simulink model "sdl_vehicle_starter"  (Simulink 7.9)
settings: Solver=ode23t  StartTime=0.0  StopTime=150  FixedStep=1e-3  RelTol=1e-4
model workspace (MAT data in the model file):
  vi = Simulink.Parameter
  vi.Value = 960
  vi.DataType = 'auto'
PreLoadFcn:
  | num_fric_surf = 6;
  | eff_tor_rad = 0.4;
  | engagement_area = 0.0025;
  | peak_normal = 0.55;
  | fric_coeff = 0.5;
  | clutchRise = 0.1;
  | velTol = 1e-3;
  | pressThresh = 0.05;
  | p0 = 20e5;
undefined symbols (not defined in the file): sigbuilder_block
libraries: fl_lib x20, nesl_utility x14, sdl_lib x12
Description:
  | Vehicle With Automatic Transmission
  | 
  | This example shows a complete vehicle with SimDriveline(TM) blocks, from
  | engine, drivetrain, and transmission, to tire and vehicle dynamics. The
  | transmission controller is preprogrammed, but can be changed to respond to
  | engine and vehicle behavior.
  | 
  | 
  | 
  | 
  | 
  | Copyright 2008-2012 The MathWorks, Inc.
CloseFcn:
  | clear num_fric_surf eff_tor_rad engagement_area
  | clear peak_normal fric_coeff clutchRise
  | clear velTol pressThresh p0
settings Model: FPTRunName=Active  Creator=MathWorks  LastModifiedBy=sbiagion  ExtModeAutoUpdateStatusClock=off
settings SolverCC: ZcThreshold=0  ZeroCrossAlgorithm=Adaptive
settings DataIOCC: SaveOutput=off  SignalLogging=off  DSMLogging=off  SaveTime=off  SignalLoggingName=logsOut
settings OptimizationCC: InitFltsAndDblsToZero=on
settings DebuggingCC: AlgebraicLoopMsg=none  SaveWithParameterizedLinksMsg=none  CheckExecutionContextPreStartOutputMsg=on  CheckExecutionContextRuntimeOutputMsg=on  SignalResolutionControl=TryResolveAllWithWarning  MaskedZcDiagnostic=none  SolverPrmCheckMsg=none  MultiTaskDSMMsg=warning  MultiTaskCondExecSysMsg=none  SigSpecEnsureSampleTimeMsg=none  StrictBusMsg=None
settings HardwareCC: TargetEndianess=LittleEndian  TargetHWDeviceType=MATLAB Host  ProdEqTarget=off
settings ModelReferenceCC: UpdateModelReferenceTargets=IfOutOfDate
settings RTWCC: ProcessScript=grt_make_rtw_hook  IncludeERTFirstTime=on
settings CodeAppCC: CustomSymbolStrType=$N$R$M_T
settings GRTTargetCC: CombineOutputUpdateFcns=off  GRTInterface=on

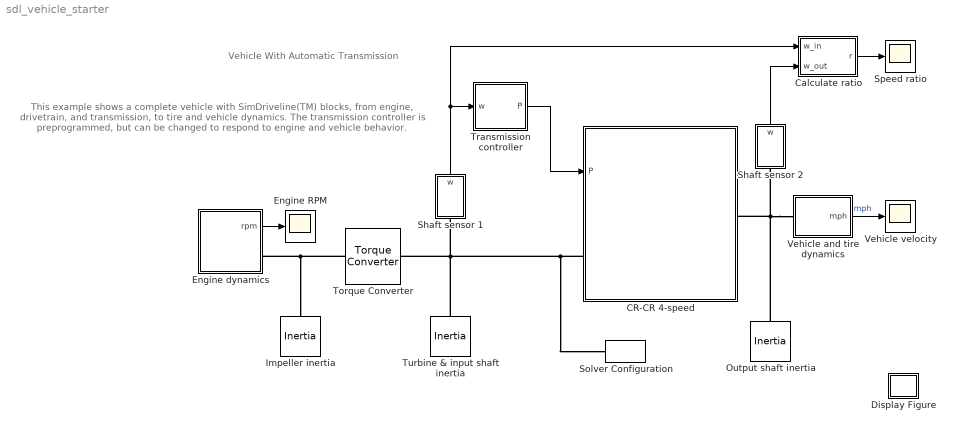
== system sdl_vehicle_starter ==
  note: Vehicle With Automatic Transmission
  note: This example shows a complete vehicle
      | with SimDriveline(TM) blocks, from
      | engine, drivetrain, and transmission, to
      | tire and vehicle dynamics. The
      | transmission controller is
      | preprogrammed, but can be changed to
      | respond to engine and vehicle behavior.
  CR-CR 4-speed : Subsystem  mask(CR-CR 4-Speed){}
      mask help: This is a template for a CR-CR 4-speed transmission. Copy it to your model, open it as a subsystem, and modify it for your use.
      mask init:
      | drive_preinitmask(); Icon = drive_crcrgearblock('Mask');
      settings: OpenFcn=open_system(gcbh,'force');
      mask Help: web(drive_help);
      mask Display:
      | plot(Icon.x1,Icon.y1);
      | plot(Icon.x1_1,Icon.y1_1);
      | plot(Icon.x2,Icon.y2);
      | plot(Icon.x3,Icon.y3);
      | plot(Icon.x3_1,Icon.y3_1);
      | plot(Icon.x4,Icon.y4);
      | plot(Icon.x5,Icon.y5);
      | plot(Icon.x6,Icon.y6);
      | plot(Icon.x7,Icon.y7);
      | plot(Icon.x8,Icon.y8);
      | plot(Icon.x9,Icon.y9);
      | plot(Icon.x10,Icon.y10);
      | plot(Icon.x11,Icon.y11);
      | plot(Icon.x12,Icon.y12);
      | plot(Icon.x13,Icon.y13);
      | plot(Icon.x14,Icon.y14);
      | plot(Icon.x15,Icon.y15);
      | plot(Icon.x16,Icon.y16);
      | plot(Icon.x16_1,Icon.y16_1);
      | plot(Icon.x16_2,Icon.y16_2);
      | plot(Icon.x17,Icon.y17);
      | plot(Icon.x18,Icon.y18);
      | plot(Icon.x18_1,Icon.y18_1);
      | plot(Icon.x18_2,Icon.y18_2);
      | plot(Icon.x19,Icon.y19);
      | plot(Icon.x20,Icon.y20);
      | plot(Icon.x21,Icon.y21);
      | plot(Icon.x22,Icon.y22);
      | plot(Icon.x23,Icon.y23);
      | plot(Icon.x24,Icon.y24);
      | plot(Icon.x25,Icon.y25);
      | plot(Icon.x26,Icon.y26);
      | plot(Icon.x27,Icon.y27);
      | plot(Icon.x28,Icon.y28);
      | plot(Icon.x29,Icon.y29);
      | 
      | plot(Icon.LowerLeftx,Icon.LowerLefty);
      | plot(Icon.UpperRightx,Icon.UpperRighty);
  Calculate ratio : Subsystem
  Display Figure : Subsystem  Description=Help callback for CR-CR transmission model: sdl_vehicle.mdl
      settings: OpenFcn=helpview([docroot '/toolbox/physmod/sdl/sdl.map'], 'sdl_vehicle_help');
      mask Type: Help callback
      mask Display: image(imread('info.bmp'))
  Engine RPM : Scope
      settings: TimeRange=150  YMin=500  YMax=4000  MaxDataPoints=500000  SampleTime=0.1
  Engine dynamics : Subsystem
  Impeller inertia : fl_lib/Mechanical/Rotational Elements/Inertia  inertia=0.02 kg*m^2  initial_velocity=vi rpm  t_Log=off  LocalVarNames=|t  LocalVarDescs=|t  LocalVarLogging=0
  Output shaft inertia : fl_lib/Mechanical/Rotational Elements/Inertia  inertia=1e-1 kg*m^2  initial_velocity=0 rad/s  t_Log=off  LocalVarNames=|t  LocalVarDescs=|t  LocalVarLogging=0
  Shaft sensor 1 : Subsystem
  Shaft sensor 2 : Subsystem
  Solver Configuration : nesl_utility/Solver Configuration  PhysicalDomain=network_engine_domain  LeftPortType=input  RightPortType=generic  SubClassName=solver  UseCustomDae=off  DoDC=off  ResidualTolerance=1e-9  UseLocalSolver=off  LocalSolverChoice=NE_BACKWARD_EULER_ADVANCER  LocalSolverSampleTime=0.001  DoFixedCost=off  MaxNonlinIter=3  MaxModeIter=2  LinearAlgebra=Sparse  Accelerate=off  Profile=off  UseLocalSampling=off  DelaysMemoryBudget=1024
  Speed ratio : Scope
      settings: TimeRange=150  YMin=0  YMax=1.5  SaveName=ScopeData5  MaxDataPoints=500000  SampleTime=0.1
  Torque Converter : sdl_lib/Couplings & Drives/Torque Converter  n_vector=[0 0.50 0.60 0.70 0.80 0.87 0.92 0.94 0.96 0.97]  trq_vector=[2.2320 1.5462 1.4058 1.2746 1.1528 1.0732 1.0192 0.9983 0.9983 0.9983]  cf_vector_parameterization=1  cf_vector_reference_speed=1  cf_vector=[12.2938 12.8588 13.1452 13.6285 14.6163 16.2675 19.3503 22.1046 29.9986 50.00] (rad/s)/(N*m)^0.5  cf_vector_sq=1e-3*[ 6.616 6.048 5.787 5.384 4.681 3.779 2.671 2.047 1.111 0.400] N*m/(rad/s)^2  interp_method=1  extrap_method=1  model_lag=0  tau=0.02 s  initial_trq_ratio=0  trq_imp_s_Log=off  trq_imp_Log=off  torque_ratio_Log=off  trq_ratio_inst_Log=off  trq_trb_Log=off  w_imp_Log=off  w_trb_Log=off  power_imp_Log=off  power_trb_Log=off  power_loss_Log=off  efficiency_Log=off  LocalVarNames=|trq_imp_s|trq_imp|N_t|trq_ratio_inst|trq_trb|w_imp|w_trb|power_imp|power_trb|power_loss|efficiency  LocalVarDescs=|Static torque on impeller shaft (N*m)|Transient torque on impeller shaft (N*m)|Static torque ratio|Instant torque ratio|Torque on turbine shaft (N*m)|Angular velocity of impeller shaft (rad/s)|Angular velocity of turbine shaft (rad/s)|Power on impeller shaft (W)|Power on turbine shaft (W)|Power loss (W)|Efficiency)  LocalVarLogging=[0 0 0 0 0 0 0 0 0 0 0]
  Transmission controller : Subsystem
  Turbine & input shaft inertia : fl_lib/Mechanical/Rotational Elements/Inertia  inertia=1e-2 kg*m^2  initial_velocity=0 rad/s  t_Log=off  LocalVarNames=|t  LocalVarDescs=|t  LocalVarLogging=0
  Vehicle velocity : Scope
      settings: YMin=0  YMax=120  SaveName=ScopeData2  MaxDataPoints=500000  SampleTime=0.1
  Vehicle and tire dynamics : Subsystem
  wires:
  Shaft sensor 1/1(w) -> Calculate ratio/1(w_in), Transmission controller/1(w)
  Transmission controller/1(P) -> CR-CR 4-speed/1(P)
  Shaft sensor 2/1(w) -> Calculate ratio/2(w_out)
  Calculate ratio/1(r) -> Speed ratio/1
  Vehicle and tire dynamics/1(mph) -> Vehicle velocity/1  "mph"
  Engine dynamics/1(rpm) -> Engine RPM/1
  connections:
  Torque Converter/RConn1 -- Shaft sensor 1/LConn1 -- Turbine & input shaft inertia/LConn1 -- CR-CR 4-speed/LConn1 -- Solver Configuration/RConn1
  Vehicle and tire dynamics/LConn1 -- Shaft sensor 2/LConn1 -- Output shaft inertia/LConn1 -- CR-CR 4-speed/RConn1
  Engine dynamics/RConn1 -- Impeller inertia/LConn1 -- Torque Converter/LConn1

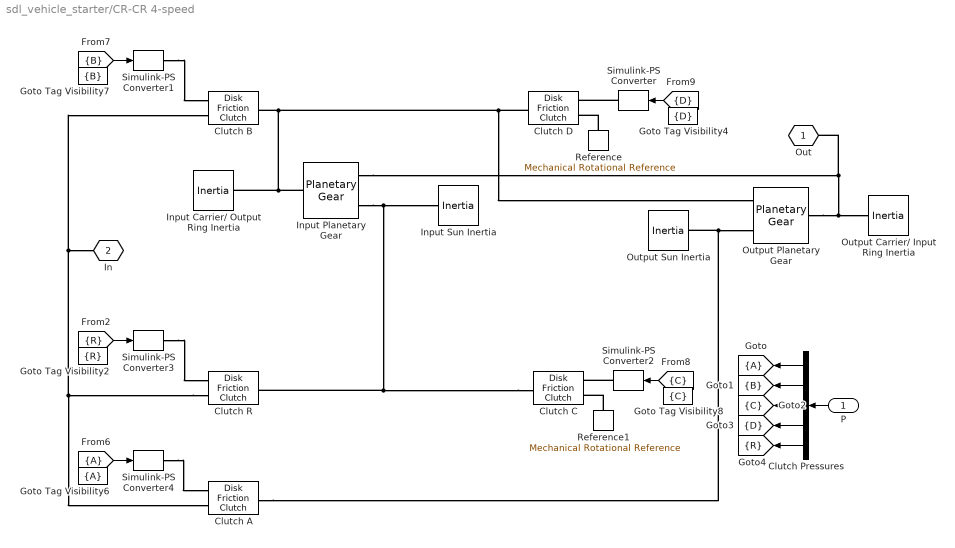
== system sdl_vehicle_starter/CR-CR 4-speed ==
  P : Inport
  Clutch Pressures : Demux  Outputs=5
  Clutch A : sdl_lib/Clutches/Disk Friction Clutch  geometry_model=1  r_eff=eff_tor_rad m  d_o=0.15 m  d_i=0.1 m  nS=num_fric_surf  piston_area=engagement_area m^2  friction_model=1  mu_coulomb=fric_coeff  mu_w_vector=[ 0 0.1 0.2 0.3 0.4 0.5 1 2 5 10 100 1000 ] rad/s  mu_coulomb_vector=[ 0.29 0.28 0.26 0.22 0.21 0.2 0.2 0.19 0.19 0.19 0.19 0.19 ]  mu_interp_method=1  mu_extrap_method=1  mu_static=peak_normal  d_f=1  w_tol=velTol rad/s  pressure_min=pressThresh*p0 Pa  mu_visc=0 N*m/(rad/s)  initial_state_locked=1  LocalVarLogging=[]
  Clutch B : sdl_lib/Clutches/Disk Friction Clutch  geometry_model=1  r_eff=eff_tor_rad m  d_o=0.15 m  d_i=0.1 m  nS=num_fric_surf  piston_area=engagement_area m^2  friction_model=1  mu_coulomb=fric_coeff  mu_w_vector=[ 0 0.1 0.2 0.3 0.4 0.5 1 2 5 10 100 1000 ] rad/s  mu_coulomb_vector=[ 0.29 0.28 0.26 0.22 0.21 0.2 0.2 0.19 0.19 0.19 0.19 0.19 ]  mu_interp_method=1  mu_extrap_method=1  mu_static=peak_normal  d_f=1  w_tol=velTol rad/s  pressure_min=pressThresh*p0 Pa  mu_visc=0 N*m/(rad/s)  initial_state_locked=0  LocalVarLogging=[]
  Clutch C : sdl_lib/Clutches/Disk Friction Clutch  geometry_model=1  r_eff=eff_tor_rad m  d_o=0.15 m  d_i=0.1 m  nS=num_fric_surf  piston_area=engagement_area m^2  friction_model=1  mu_coulomb=fric_coeff  mu_w_vector=[ 0 0.1 0.2 0.3 0.4 0.5 1 2 5 10 100 1000 ] rad/s  mu_coulomb_vector=[ 0.29 0.28 0.26 0.22 0.21 0.2 0.2 0.19 0.19 0.19 0.19 0.19 ]  mu_interp_method=1  mu_extrap_method=1  mu_static=peak_normal  d_f=1  w_tol=velTol rad/s  pressure_min=pressThresh*p0 Pa  mu_visc=0 N*m/(rad/s)  initial_state_locked=0  LocalVarLogging=[]
  Clutch D : sdl_lib/Clutches/Disk Friction Clutch  geometry_model=1  r_eff=eff_tor_rad m  d_o=0.15 m  d_i=0.1 m  nS=num_fric_surf  piston_area=engagement_area m^2  friction_model=1  mu_coulomb=fric_coeff  mu_w_vector=[ 0 0.1 0.2 0.3 0.4 0.5 1 2 5 10 100 1000 ] rad/s  mu_coulomb_vector=[ 0.29 0.28 0.26 0.22 0.21 0.2 0.2 0.19 0.19 0.19 0.19 0.19 ]  mu_interp_method=1  mu_extrap_method=1  mu_static=peak_normal  d_f=1  w_tol=velTol rad/s  pressure_min=pressThresh*p0 Pa  mu_visc=0 N*m/(rad/s)  initial_state_locked=1  LocalVarLogging=[]
  Clutch R : sdl_lib/Clutches/Disk Friction Clutch  geometry_model=1  r_eff=eff_tor_rad m  d_o=0.15 m  d_i=0.1 m  nS=num_fric_surf  piston_area=engagement_area m^2  friction_model=1  mu_coulomb=fric_coeff  mu_w_vector=[ 0 0.1 0.2 0.3 0.4 0.5 1 2 5 10 100 1000 ] rad/s  mu_coulomb_vector=[ 0.29 0.28 0.26 0.22 0.21 0.2 0.2 0.19 0.19 0.19 0.19 0.19 ]  mu_interp_method=1  mu_extrap_method=1  mu_static=peak_normal  d_f=1  w_tol=velTol rad/s  pressure_min=pressThresh*p0 Pa  mu_visc=0 N*m/(rad/s)  initial_state_locked=0  LocalVarLogging=[]
  Goto Tag Visibility2 : GotoTagVisibility  GotoTag=R
  Goto Tag Visibility4 : GotoTagVisibility  GotoTag=D
  Goto Tag Visibility6 : GotoTagVisibility
  Goto Tag Visibility7 : GotoTagVisibility  GotoTag=B
  Goto Tag Visibility8 : GotoTagVisibility  GotoTag=C
  "Input Planetary Gear " : sdl_lib/Gears/Planetary Gear  rs_ratio=2.2258  friction_model=1  efficiency=[ 0.96 0.98 ]  mu_visc=[ 0 0 ] N*m/(rad/s)  w_thr=[ 0.01 0.01 ] rad/s  LocalVarLogging=[]
  Input Sun Inertia : fl_lib/Mechanical/Rotational Elements/Inertia  inertia=1e-4 kg*m^2  initial_velocity=0 rad/s  t_Log=off  LocalVarNames=|t  LocalVarDescs=|t  LocalVarLogging=0
  Input Carrier/ Output Ring Inertia : fl_lib/Mechanical/Rotational Elements/Inertia  inertia=1e-4 kg*m^2  initial_velocity=0 rad/s  t_Log=off  LocalVarNames=|t  LocalVarDescs=|t  LocalVarLogging=0
  Output Planetary Gear : sdl_lib/Gears/Planetary Gear  rs_ratio=1.84  friction_model=1  efficiency=[ 0.96 0.98 ]  mu_visc=[0 0] N*m/(rad/s)  w_thr=[ 0.01 0.01 ] rad/s  LocalVarLogging=[]
  Output Sun Inertia : fl_lib/Mechanical/Rotational Elements/Inertia  inertia=1e-4 kg*m^2  initial_velocity=0 rad/s  t_Log=off  LocalVarNames=|t  LocalVarDescs=|t  LocalVarLogging=0
  "Output Carrier/ Input Ring Inertia " : fl_lib/Mechanical/Rotational Elements/Inertia  inertia=1e-4 kg*m^2  initial_velocity=0 rad/s  t_Log=off  LocalVarNames=|t  LocalVarDescs=|t  LocalVarLogging=0
  Reference : fl_lib/Mechanical/Rotational Elements/Mechanical Rotational Reference  t_Log=off  LocalVarNames=|t  LocalVarDescs=|t  LocalVarLogging=0
  Reference1 : fl_lib/Mechanical/Rotational Elements/Mechanical Rotational Reference  t_Log=off  LocalVarNames=|t  LocalVarDescs=|t  LocalVarLogging=0
  Simulink-PS Converter{,1..4} (5 alike) : nesl_utility/Simulink-PS Converter  PhysicalDomain=network_engine_domain  LeftPortType=input  RightPortType=output  SubClassName=ps_input  Unit=1  AffineConversion=off  InputFilterTimeConstant=.001  UdotUserProvided=0  SimscapeFilterOrder=1  InputFiltering=off
  Out : PMIOPort  Tag=PMCPort  Port=1  Side=Right
  In : PMIOPort  Tag=PMCPort  Port=2  Side=Left
  tag scope: A=scoped, B=scoped, C=scoped, D=scoped, R=scoped
  wires:
  [A] -> Simulink-PS Converter4/1
  [R] -> Simulink-PS Converter3/1
  [C] -> Simulink-PS Converter2/1
  [B] -> Simulink-PS Converter1/1
  [D] -> Simulink-PS Converter/1
  Clutch Pressures/5 -> [R]
  Clutch Pressures/4 -> [D]
  Clutch Pressures/3 -> [C]
  Clutch Pressures/2 -> [B]
  Clutch Pressures/1 -> [A]
  P/1 -> Clutch Pressures/1
  connections:
  Simulink-PS Converter4/RConn1 -- Clutch A/LConn1
  Simulink-PS Converter3/RConn1 -- Clutch R/LConn1
  Simulink-PS Converter2/RConn1 -- Clutch C/LConn1
  Reference1/LConn1 -- Clutch C/LConn2
  Clutch R/LConn2 -- Clutch B/LConn2 -- In/RConn1 -- Clutch A/LConn2
  Simulink-PS Converter1/RConn1 -- Clutch B/LConn1
  Input Carrier/ Output Ring Inertia/LConn1 -- "Input Planetary Gear "/LConn1 -- Clutch D/RConn1 -- Output Planetary Gear/RConn1 -- Clutch B/RConn1
  Clutch C/RConn1 -- Input Sun Inertia/LConn1 -- "Input Planetary Gear "/RConn2 -- Clutch R/RConn1
  Simulink-PS Converter/RConn1 -- Clutch D/LConn1
  Reference/LConn1 -- Clutch D/LConn2
  Output Sun Inertia/LConn1 -- Output Planetary Gear/RConn2 -- Clutch A/RConn1
  Out/RConn1 -- "Output Carrier/ Input Ring Inertia "/LConn1 -- Output Planetary Gear/LConn1 -- "Input Planetary Gear "/RConn1

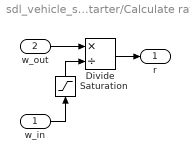
== system sdl_vehicle_starter/Calculate ratio ==
  w_in : Inport
  w_out : Inport  Port=2
  Divide : Product  Inputs=*/
  Saturation : Saturate  UpperLimit=inf  LowerLimit=0.001  ZeroCross=off
  r : Outport
  wires:
  Saturation/1 -> Divide/2
  w_in/1 -> Saturation/1
  w_out/1 -> Divide/1
  Divide/1 -> r/1

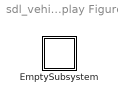
== system sdl_vehicle_starter/Display Figure ==
  EmptySubsystem : Subsystem

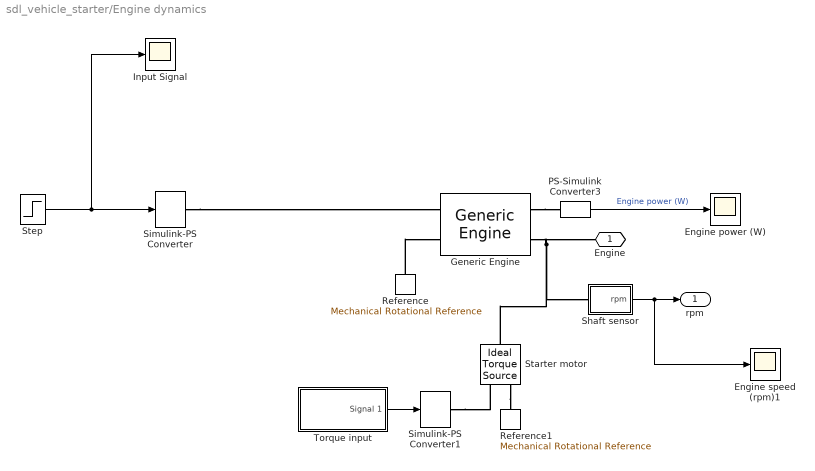
== system sdl_vehicle_starter/Engine dynamics ==
  Engine power (W) : Scope
      settings: TimeRange=150  YMin=-50000  YMax=150000  MaxDataPoints=500000  SampleTime=0.1
  Engine speed (rpm)1 : Scope
      settings: TimeRange=150  YMin=0  YMax=4000  SaveName=ScopeData6  MaxDataPoints=500000  SampleTime=0.1
  Generic Engine : sdl_lib/Engines/Generic Engine  model_parameterization=1  engine_type=1  P_max=1.5e+5 W  w_P_max=4.5e+3 rpm  w_max=6e+3 rpm  w_min=500 rpm  w_tab=[ 500 1000 2e+3 3e+3 4e+3 5e+3 6e+3 7e+3 ] rpm  trq_tab=[ 380 380 380 380 350 280 200 80 ] N*m  pwr_tab=[ 2e+4 4e+4 7.8e+4 1.2e+5 1.45e+5 1.48e+5 1.25e+5 6e+4 ] W  interp_method=1  model_inertia=1  inertia=0.08 kg*m^2  initial_velocity=vi rpm  model_time_constant=1  time_constant=0.4 s  T0=0  w_thr=100 rpm  LocalVarLogging=[]
  Input Signal : Scope
      settings: TimeRange=150  YMin=-0.5  YMax=1.5  SaveName=ScopeData3  MaxDataPoints=500000  SampleTime=0.1
  PS-Simulink Converter3 : nesl_utility/PS-Simulink Converter  PhysicalDomain=network_engine_domain  LeftPortType=input  RightPortType=output  SubClassName=ps_output  Unit=W  AffineConversion=off
  Reference : fl_lib/Mechanical/Rotational Elements/Mechanical Rotational Reference  t_Log=off  LocalVarNames=|t  LocalVarDescs=|t  LocalVarLogging=0
  Reference1 : fl_lib/Mechanical/Rotational Elements/Mechanical Rotational Reference  t_Log=off  LocalVarNames=|t  LocalVarDescs=|t  LocalVarLogging=0
  Shaft sensor : Subsystem
  Simulink-PS Converter1 : nesl_utility/Simulink-PS Converter  PhysicalDomain=network_engine_domain  LeftPortType=input  RightPortType=output  SubClassName=ps_input  Unit=1  AffineConversion=off  InputFilterTimeConstant=0.001  UdotUserProvided=1  SimscapeFilterOrder=1  InputFiltering=on
  Simulink-PS Converter : nesl_utility/Simulink-PS Converter  PhysicalDomain=network_engine_domain  LeftPortType=input  RightPortType=output  SubClassName=ps_input  Unit=1  AffineConversion=off  InputFilterTimeConstant=.001  UdotUserProvided=[]  SimscapeFilterOrder=1  InputFiltering=off
  Starter motor : fl_lib/Mechanical/Mechanical Sources/Ideal Torque Source  w_Log=off  t_Log=off  LocalVarNames=|w|t  LocalVarDescs=|w|t  LocalVarLogging=[0 0]
  Step : Step  Time=60  SampleTime=0
  Torque input : Subsystem  Tag=STV Subsys  LoadFcn=sigbuilder_block('load');  StartFcn=sigbuilder_block('start');  StopFcn=sigbuilder_block('stop');  ClipboardFcn=sigbuilder_block('clipboard');  mask(Sigbuilder block){}
      mask help: Simulink:masks:SigbuilderBlock_MD
      mask init:
      | if ~strcmp(get_param(bdroot(gcbh),'SimulationStatus'),'stopped') tuvar = sigbuilder_block('maskInit'); end
      settings: CopyFcn=sigbuilder_block('copy');  DeleteFcn=sigbuilder_block('delete');  ModelCloseFcn=sigbuilder_block('modelClose');  PreSaveFcn=sigbuilder_block('preSave');  PauseFcn=sigbuilder_block('pause');  ContinueFcn=sigbuilder_block('continue');  NameChangeFcn=sigbuilder_block('namechange');  OpenFcn=sigbuilder_block('open',[69 114 550.5 399.75 ]);  CloseFcn=sigbuilder_block('close');
      mask Display: plot(0, 0, 100, 100,[2, 2, 32, 32, 2], [68, 8, 8, 68, 68],[32, 2], [38, 38], [32, 19, 2],[53, 60, 44], [32, 17, 17, 2],[16, 16, 31, 31]);txt = getActiveGroup(gcbh);text(2, 100, txt,'verticalAlignment', 'top');
  Engine : PMIOPort  Port=1  Side=Right
  rpm : Outport
  wires:
  PS-Simulink Converter3/1 -> Engine power (W)/1  "Engine power (W)"
  Step/1 -> Input Signal/1, Simulink-PS Converter/1
  Shaft sensor/1(rpm) -> Engine speed (rpm)1/1, rpm/1
  Torque input/1(Signal 1) -> Simulink-PS Converter1/1
  connections:
  Reference/LConn1 -- Generic Engine/LConn2
  Generic Engine/RConn1 -- PS-Simulink Converter3/LConn1
  Generic Engine/RConn2 -- Engine/RConn1 -- Starter motor/LConn1 -- Shaft sensor/LConn1
  Simulink-PS Converter1/RConn1 -- Starter motor/RConn1
  Starter motor/RConn2 -- Reference1/LConn1
  Simulink-PS Converter/RConn1 -- Generic Engine/LConn1

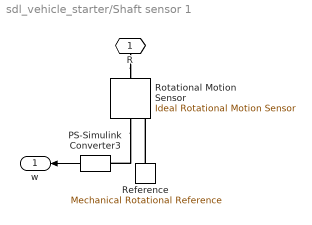
== system sdl_vehicle_starter/Shaft sensor 1 ==
  PS-Simulink Converter3 : nesl_utility/PS-Simulink Converter  PhysicalDomain=network_engine_domain  LeftPortType=input  RightPortType=output  SubClassName=ps_output  Unit=rad/s  AffineConversion=off
  Reference : fl_lib/Mechanical/Rotational Elements/Mechanical Rotational Reference  t_Log=off  LocalVarNames=|t  LocalVarDescs=|t  LocalVarLogging=0
  Rotational Motion Sensor : fl_lib/Mechanical/Mechanical Sensors/Ideal Rotational Motion Sensor  offset=0 rad  w_Log=off  t_Log=off  phi_Log=off  LocalVarNames=|w|t|phi  LocalVarDescs=|w|t|phi  LocalVarLogging=[0 0 0]
  R : PMIOPort  Port=1  Side=Left
  w : Outport
  wires:
  PS-Simulink Converter3/1 -> w/1
  connections:
  R/RConn1 -- Rotational Motion Sensor/LConn1
  Reference/LConn1 -- Rotational Motion Sensor/RConn1
  Rotational Motion Sensor/RConn2 -- PS-Simulink Converter3/LConn1

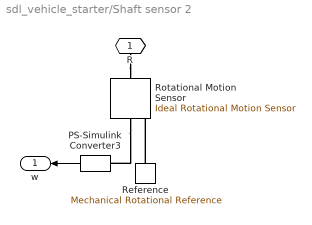
== system sdl_vehicle_starter/Shaft sensor 2 ==
  PS-Simulink Converter3 : nesl_utility/PS-Simulink Converter  PhysicalDomain=network_engine_domain  LeftPortType=input  RightPortType=output  SubClassName=ps_output  Unit=1  AffineConversion=off
  Reference : fl_lib/Mechanical/Rotational Elements/Mechanical Rotational Reference  t_Log=off  LocalVarNames=|t  LocalVarDescs=|t  LocalVarLogging=0
  Rotational Motion Sensor : fl_lib/Mechanical/Mechanical Sensors/Ideal Rotational Motion Sensor  offset=0 rad  w_Log=off  t_Log=off  phi_Log=off  LocalVarNames=|w|t|phi  LocalVarDescs=|w|t|phi  LocalVarLogging=[0 0 0]
  R : PMIOPort  Port=1  Side=Left
  w : Outport
  wires:
  PS-Simulink Converter3/1 -> w/1
  connections:
  Rotational Motion Sensor/RConn2 -- PS-Simulink Converter3/LConn1
  Reference/LConn1 -- Rotational Motion Sensor/RConn1
  R/RConn1 -- Rotational Motion Sensor/LConn1

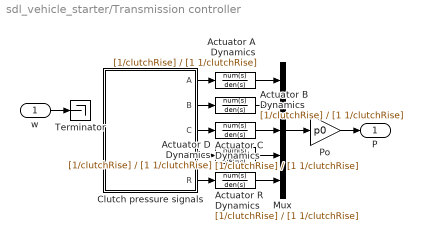
== system sdl_vehicle_starter/Transmission controller ==
  w : Inport
  Actuator A Dynamics : TransferFcn  Numerator=[1/clutchRise]  Denominator=[1 1/clutchRise]
  Actuator B Dynamics : TransferFcn  Numerator=[1/clutchRise]  Denominator=[1 1/clutchRise]
  Actuator C Dynamics : TransferFcn  Numerator=[1/clutchRise]  Denominator=[1 1/clutchRise]
  Actuator D Dynamics : TransferFcn  Numerator=[1/clutchRise]  Denominator=[1 1/clutchRise]
  Actuator R Dynamics : TransferFcn  Numerator=[1/clutchRise]  Denominator=[1 1/clutchRise]
  Clutch pressure signals : Subsystem  Tag=STV Subsys  LoadFcn=sigbuilder_block('load');  StartFcn=sigbuilder_block('start');  StopFcn=sigbuilder_block('stop');  ClipboardFcn=sigbuilder_block('clipboard');  mask(Sigbuilder block){}
      mask help: Sigbuilder GUI
      mask init:
      | if ~strcmp(get_param(bdroot(gcbh),'SimulationStatus'),'stopped') tuvar = sigbuilder_block('maskInit'); end
      settings: CopyFcn=sigbuilder_block('copy');  DeleteFcn=sigbuilder_block('delete');  ModelCloseFcn=sigbuilder_block('modelClose');  PreSaveFcn=sigbuilder_block('preSave');  PauseFcn=sigbuilder_block('pause')  ContinueFcn=sigbuilder_block('continue')  NameChangeFcn=sigbuilder_block('namechange');  OpenFcn=sigbuilder_block('open',[35.25 309 504 456.75 ]);  CloseFcn=sigbuilder_block('close');
      mask Display: plot(0, 0, 100, 100,[2, 2, 32, 32, 2], [68, 8, 8, 68, 68],[32, 2], [38, 38], [32, 19, 2],[53, 60, 44], [32, 17, 17, 2],[16, 16, 31, 31]);txt = getActiveGroup(gcbh);,text(2, 88, txt);
  Mux : Mux  Inputs=5
  Po : Gain  Gain=p0
  Terminator : Terminator
  P : Outport
  wires:
  Clutch pressure signals/5(R) -> Actuator R Dynamics/1
  Actuator R Dynamics/1 -> Mux/5
  Actuator C Dynamics/1 -> Mux/3
  Actuator B Dynamics/1 -> Mux/2
  Clutch pressure signals/4(D) -> Actuator D Dynamics/1
  Clutch pressure signals/3(C) -> Actuator C Dynamics/1
  Clutch pressure signals/2(B) -> Actuator B Dynamics/1
  Clutch pressure signals/1(A) -> Actuator A Dynamics/1
  Mux/1 -> Po/1
  w/1 -> Terminator/1
  Po/1 -> P/1
  Actuator A Dynamics/1 -> Mux/1
  Actuator D Dynamics/1 -> Mux/4

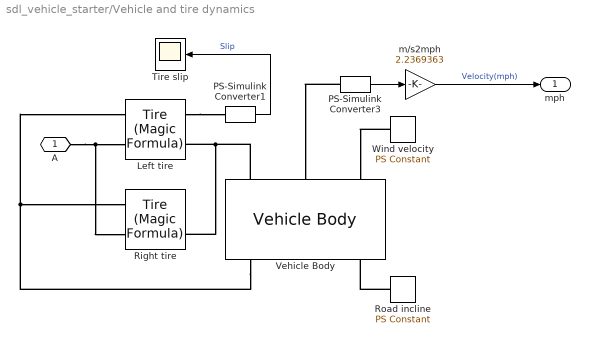
== system sdl_vehicle_starter/Vehicle and tire dynamics ==
  Left tire : sdl_lib/Tires & Vehicles/Tire (Magic Formula)  parameterization=1  F_z1=3000 N  F_x1=3500 N  kappa1=10  B_m=10  C_m=1.9  D_m=1  E_m=0.97  fz0=4e+3 N  p_Cx=1.685  p_Dx=[ 1.21 -0.037 ]  p_Ex=[ 0.344 0.095 -0.02 0 ]  p_Kx=[ 21.51 -0.163 0.245 ]  p_Hx=[ -0.002 0.002 ]  p_Vx=[ 0 0 ]  v_tr_thr=0.1 m/s  r_e=0.3 m  model_compliance=0  stiffness=1e+6 N/m  damping=1000 N/(m/s)  model_inertia=1  inertia=1e-2 kg*m^2  initial_velocity=0 rpm  LocalVarLogging=[]
  PS-Simulink Converter1 : nesl_utility/PS-Simulink Converter  PhysicalDomain=network_engine_domain  LeftPortType=input  RightPortType=output  SubClassName=ps_output  Unit=1  AffineConversion=off
  PS-Simulink Converter3 : nesl_utility/PS-Simulink Converter  PhysicalDomain=network_engine_domain  LeftPortType=input  RightPortType=output  SubClassName=ps_output  Unit=m/s  AffineConversion=off
  Right tire : sdl_lib/Tires & Vehicles/Tire (Magic Formula)  parameterization=1  F_z1=3000 N  F_x1=3500 N  kappa1=10  B_m=10  C_m=1.9  D_m=1  E_m=0.97  fz0=4e+3 N  p_Cx=1.685  p_Dx=[ 1.21 -0.037 ]  p_Ex=[ 0.344 0.095 -0.02 0 ]  p_Kx=[ 21.51 -0.163 0.245 ]  p_Hx=[ -0.002 0.002 ]  p_Vx=[ 0 0 ]  v_tr_thr=0.1 m/s  r_e=0.3 m  model_compliance=0  stiffness=1e+6 N/m  damping=1000 N/(m/s)  model_inertia=1  inertia=1e-2 kg*m^2  initial_velocity=0 rpm  LocalVarLogging=[]
  Road incline : fl_lib/Physical Signals/Sources/PS Constant  constant=0  LocalVarLogging=[]
  Tire slip : Scope
      settings: YMin=0  YMax=0.1  SaveName=ScopeData4  MaxDataPoints=500000  SampleTime=0.1
  Vehicle Body : sdl_lib/Tires & Vehicles/Vehicle Body  mass=1200 kg  n_w=2  x_f=1.4 m  x_r=1.6 m  y_c=0.5 m  area=3 m^2  Cd=0.4  v0=0 m/s  g=9.81 m/s^2  rho=1.18 kg/m^3  v_Log=off  f_Log=off  LocalVarNames=|v|f  LocalVarDescs=|v|f  LocalVarLogging=[0 0]
  Wind velocity : fl_lib/Physical Signals/Sources/PS Constant  constant=5  LocalVarLogging=[]
  m/s2mph : Gain  Gain=2.2369363
  A : PMIOPort  Port=1  Side=Left
  mph : Outport
  wires:
  PS-Simulink Converter3/1 -> m/s2mph/1
  m/s2mph/1 -> mph/1  "Velocity(mph)"
  PS-Simulink Converter1/1 -> Tire slip/1  "Slip"
  connections:
  Road incline/RConn1 -- Vehicle Body/RConn3
  Wind velocity/RConn1 -- Vehicle Body/LConn3
  PS-Simulink Converter3/LConn1 -- Vehicle Body/LConn2
  Vehicle Body/LConn1 -- Left tire/RConn2 -- Right tire/RConn2
  Vehicle Body/RConn1 -- Left tire/LConn1 -- Right tire/LConn1
  A/RConn1 -- Left tire/LConn2 -- Right tire/LConn2
  Left tire/RConn1 -- PS-Simulink Converter1/LConn1

== system sdl_vehicle_starter/Display Figure/EmptySubsystem ==

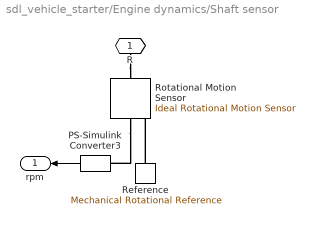
== system sdl_vehicle_starter/Engine dynamics/Shaft sensor ==
  PS-Simulink Converter3 : nesl_utility/PS-Simulink Converter  PhysicalDomain=network_engine_domain  LeftPortType=input  RightPortType=output  SubClassName=ps_output  Unit=rpm  AffineConversion=off
  Reference : fl_lib/Mechanical/Rotational Elements/Mechanical Rotational Reference  t_Log=off  LocalVarNames=|t  LocalVarDescs=|t  LocalVarLogging=0
  Rotational Motion Sensor : fl_lib/Mechanical/Mechanical Sensors/Ideal Rotational Motion Sensor  offset=0 rad  w_Log=off  t_Log=off  phi_Log=off  LocalVarNames=|w|t|phi  LocalVarDescs=|w|t|phi  LocalVarLogging=[0 0 0]
  R : PMIOPort  Port=1  Side=Left
  rpm : Outport
  wires:
  PS-Simulink Converter3/1 -> rpm/1
  connections:
  Rotational Motion Sensor/RConn2 -- PS-Simulink Converter3/LConn1
  Reference/LConn1 -- Rotational Motion Sensor/RConn1
  R/RConn1 -- Rotational Motion Sensor/LConn1

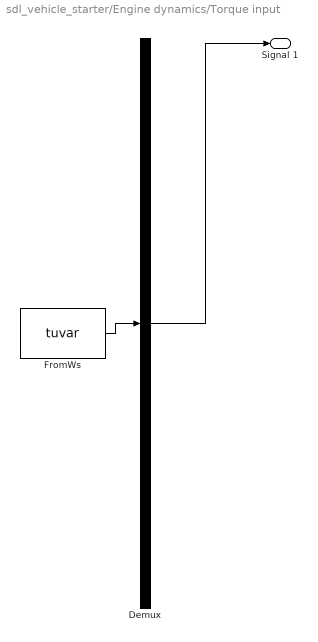
== system sdl_vehicle_starter/Engine dynamics/Torque input ==
  Demux : Demux  Tag=STV Demux  Outputs=1
  FromWs : FromWorkspace  Tag=STV FromWs  VariableName=tuvar  SampleTime=0  SigBuilderData=DataTag1  VnvData=DataTag2
      SigBuilderData=|
      | common.afterFinalStr = 'Extrapolate'
      | common.sampleTime = 0
      | dataSet.timeRange = [0 150]
      | dataSet.name = 'Group 1'
      | sbobj.Groups.Name = 'Group 1'
      | sbobj.Groups.Signals.Name = 'Signal 1'
      | sbobj.Groups.Signals.XData = [0 90 90 95 95 150]
      | sbobj.Groups.Signals.YData = [0 0 20 20 0 0]
      | sbobj.Groups.TimeRange = [0 150]
  Signal 1 : Outport  Tag=STV Outport
  wires:
  Demux/1 -> Signal 1/1
  FromWs/1 -> Demux/1

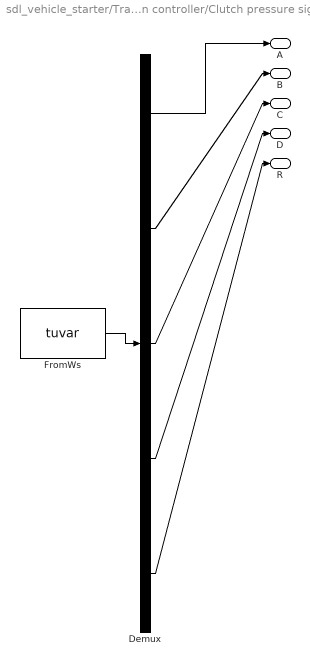
== system sdl_vehicle_starter/Transmission controller/Clutch pressure signals ==
  Demux : Demux  Tag=STV Demux  Outputs=5
  FromWs : FromWorkspace  Tag=STV FromWs  VariableName=tuvar  SampleTime=0  SigBuilderData=DataTag3  VnvData=DataTag4
      SigBuilderData=|
      | dataSet.timeRange = [0 100]
      | dataSet.name = 'Group 1'
      | sbobj.Groups.Name = 'Group 1'
      | sbobj.Groups.Signals(1).Name = 'A'
      | sbobj.Groups.Signals(1).XData = [0 0.1 75 75 100]
      | sbobj.Groups.Signals(1).YData = [1 1 1 0 0]
      | sbobj.Groups.Signals(2).Name = 'B'
      | sbobj.Groups.Signals(2).XData = [0 5 5 35 35 100]
      | sbobj.Groups.Signals(2).YData = [0 0 0 0 1 1]
      | sbobj.Groups.Signals(3).Name = 'C'
      | sbobj.Groups.Signals(3).XData = [0 10 10 10 11 15 25 35 35 43.1 75 75 100]
      | sbobj.Groups.Signals(3).YData = [0 0 0 1 1 1 1 1 0 0 0 1 1]
      | sbobj.Groups.Signals(4).Name = 'D'
      | sbobj.Groups.Signals(4).XData = [0 0.1 0.1 10 10 10 15 100]
      | sbobj.Groups.Signals(4).YData = [0 0 1 1 1 0 0 0]
      | sbobj.Groups.Signals(5).Name = 'R'
      | sbobj.Groups.Signals(5).XData = [0 100]
      | sbobj.Groups.Signals(5).YData = [0 0]
      | sbobj.Groups.TimeRange = [0 100]
  A : Outport  Tag=STV Outport
  B : Outport  Tag=STV Outport  Port=2
  C : Outport  Tag=STV Outport  Port=3
  D : Outport  Tag=STV Outport  Port=4
  R : Outport  Tag=STV Outport  Port=5
  wires:
  Demux/5 -> R/1
  Demux/1 -> A/1
  FromWs/1 -> Demux/1
  Demux/2 -> B/1
  Demux/3 -> C/1
  Demux/4 -> D/1
